simulink model "non_linear_model_2021b"  (R2021b)
settings: Solver=VariableStepAuto  StartTime=0.0  StopTime=8  MaxStep=1e-4  RelTol=1e-7
values from neighbouring files (symbols this model uses):
  beta = 20    [main.m]
undefined symbols (not defined in the file or in its folder): initial_conds, pod
libraries: shared6dof x1
settings Model: Creator=Ferran  LastModifiedBy=ferrandeandres

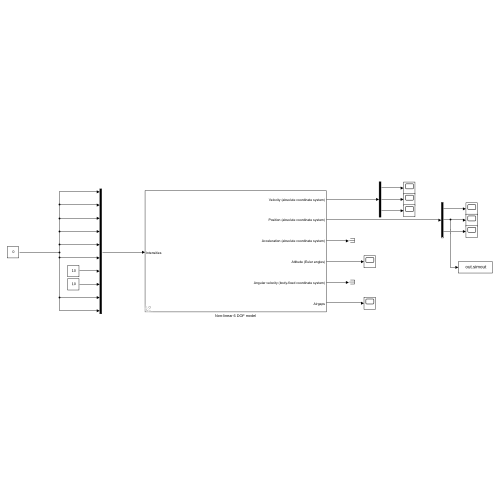
[thumbnail: Simulink's stored preview of the top-level diagram]
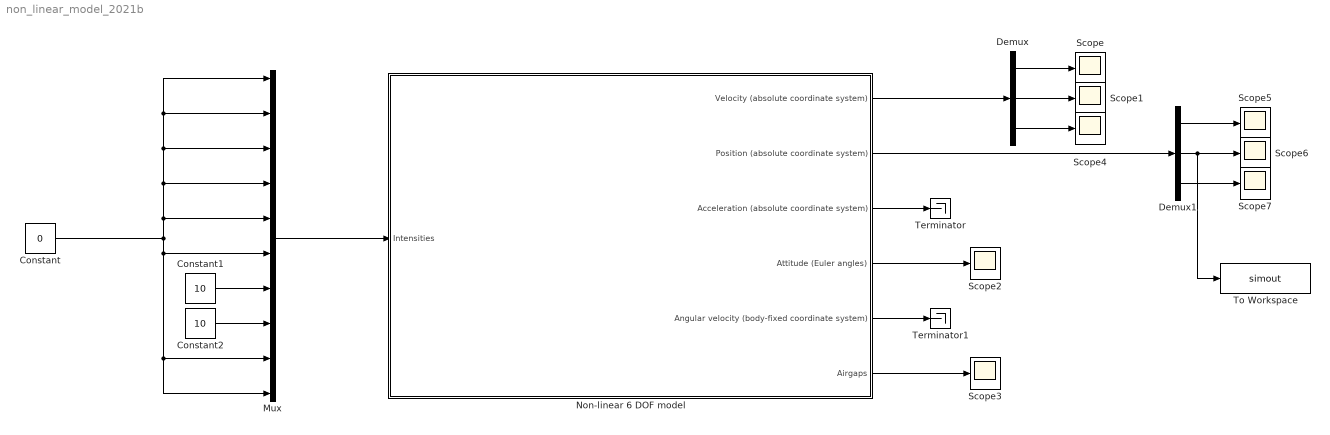
== system non_linear_model_2021b ==
  Constant : Constant  Value=0
  Constant1 : Constant  Value=10
  Constant2 : Constant  Value=10
  Demux : Demux  Outputs=3
  Demux1 : Demux  Outputs=3
  Mux : Mux  Inputs=10
  Non-linear 6 DOF model : Subsystem  AncestorBlock=libH7_6DOF/Non-linear 6 DOF model
  Scope{,1..7} (8 alike) : Scope
  Terminator : Terminator
  Terminator1 : Terminator
  To Workspace : ToWorkspace  VariableName=simout  SaveFormat=Timeseries  SampleTime=-1
  wires:
  Mux/1 -> Non-linear 6 DOF model/1(Intensities)
  Constant/1 -> Mux/4, Mux/2, Mux/1, Mux/3, Mux/5, Mux/6, Mux/9, Mux/10
  Non-linear 6 DOF model/4(Attitude (Euler angles)) -> Scope2/1
  Non-linear 6 DOF model/6(Airgaps) -> Scope3/1
  Non-linear 6 DOF model/3(Acceleration (absolute coordinate system)) -> Terminator/1
  Non-linear 6 DOF model/5(Angular velocity (body-fixed coordinate system)) -> Terminator1/1
  Non-linear 6 DOF model/1(Velocity (absolute coordinate system)) -> Demux/1
  Non-linear 6 DOF model/2(Position (absolute coordinate system)) -> Demux1/1
  Demux/1 -> Scope/1
  Demux/2 -> Scope1/1
  Demux/3 -> Scope4/1
  Demux1/1 -> Scope5/1
  Demux1/2 -> To Workspace/1, Scope6/1
  Demux1/3 -> Scope7/1
  Constant1/1 -> Mux/7
  Constant2/1 -> Mux/8

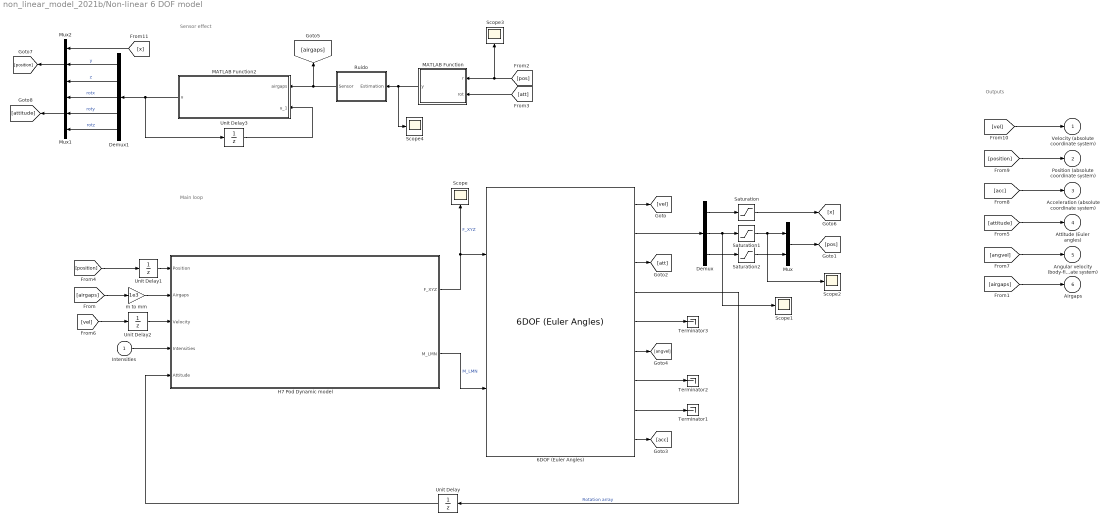
== system non_linear_model_2021b/Non-linear 6 DOF model ==
  note: Outputs
  note: Main loop
  note: Sensor effect
  Intensities : Inport
  6DOF (Euler Angles) : shared6dof/6DOF (Euler Angles)  units=Metric (MKS)  mtype=Fixed  rep=Euler Angles  xme_0=initial_conds.x_0  Vm_0=initial_conds.v_0  eul_0=initial_conds.ang_0  pm_0=initial_conds.w_0  mass_0=pod.mass.mass  mass_e=0.5  mass_f=2.0  inertia=pod.mass.inertia  inertia_e=eye(3)  inertia_f=2*eye(3)  k_quat=1.0  vre_flag=on  abi_flag=on  aMode=0  xme_statename=''  Vm_statename=''  eul_statename=''  quat_statename=''  pm_statename=''  mass_statename=''
      link override Abi: Port=9
      settings: SourceProductBaseCode=AE,PW,DR,MT,VE
  Demux : Demux  Outputs=3
  Demux1 : Demux  Outputs=5
  H7 Pod Dynamic model : Subsystem  AncestorBlock=libH7_6DOF/H7 Pod Dynamic model
      mask Display: image('FBD.png', [0.12 0.12 0.78 0.78]); % Use "Edit Image" on toolstrip to change.
  MATLAB Function : MATLAB Function  TreatAsAtomicUnit=on
  MATLAB Function2 : MATLAB Function  TreatAsAtomicUnit=on
  Mux : Mux  Inputs=2
  Mux1 : Mux  Inputs=3
  Mux2 : Mux  Inputs=3
  Ruido : Subsystem
  Saturation : Saturate  UpperLimit=20  LowerLimit=0
  Saturation1 : Saturate  UpperLimit=0.002  LowerLimit=-0.002
  Saturation2 : Saturate  UpperLimit=0.3504  LowerLimit=0.3384
  Scope{,1..4} (5 alike) : Scope
  Terminator1 : Terminator
  Terminator2 : Terminator
  Terminator3 : Terminator
  Unit Delay : UnitDelay  InitialCondition=eye(3,3)  SampleTime=-1  HasFrameUpgradeWarning=on
  Unit Delay1 : UnitDelay  InitialCondition=initial_conds.x_0  SampleTime=-1  HasFrameUpgradeWarning=on
  Unit Delay2 : UnitDelay  InitialCondition=initial_conds.v_0  SampleTime=-1  HasFrameUpgradeWarning=on
  Unit Delay3 : UnitDelay  SampleTime=-1  HasFrameUpgradeWarning=on
  m to mm : Gain  Gain=1e3
  Velocity (absolute coordinate system) : Outport
  Position (absolute coordinate system) : Outport  Port=2
  Acceleration (absolute coordinate system) : Outport  Port=3
  Attitude (Euler angles) : Outport  Port=4
  Angular velocity (body-fixed coordinate system) : Outport  Port=5
  Airgaps : Outport  Port=6
  wires:
  6DOF (Euler Angles)/7 -> Terminator2/1
  6DOF (Euler Angles)/5 -> Terminator3/1
  6DOF (Euler Angles)/8 -> Terminator1/1
  H7 Pod Dynamic model/2(M_LMN) -> 6DOF (Euler Angles)/2  "M_LMN"
  H7 Pod Dynamic model/1(F_XYZ) -> Scope/1, 6DOF (Euler Angles)/1  "F_XYZ"
  6DOF (Euler Angles)/4 -> Unit Delay/1  "Rotation array"
  Intensities/1 -> H7 Pod Dynamic model/4(Intensities)
  [vel] -> Velocity (absolute coordinate system)/1
  [attitude] -> Attitude (Euler angles)/1
  [angvel] -> Angular velocity (body-fixed coordinate system)/1
  [acc] -> Acceleration (absolute coordinate system)/1
  [position] -> Position (absolute coordinate system)/1
  [airgaps] -> Airgaps/1
  Unit Delay/1 -> H7 Pod Dynamic model/5(Attitude)
  Unit Delay1/1 -> H7 Pod Dynamic model/1(Position)
  [airgaps] -> m to mm/1
  Demux/2 -> Scope1/1, Saturation1/1
  Demux/1 -> Saturation/1
  6DOF (Euler Angles)/2 -> Demux/1
  Demux/3 -> Saturation2/1
  6DOF (Euler Angles)/3 -> [att]
  6DOF (Euler Angles)/1 -> [vel]
  6DOF (Euler Angles)/9 -> [acc]
  6DOF (Euler Angles)/6 -> [angvel]
  [pos] -> Scope3/1, MATLAB Function/1(r)
  [att] -> MATLAB Function/2(rot)
  MATLAB Function/1(y) -> Scope4/1, Ruido/1(Estimation)
  Ruido/1(Sensor) -> MATLAB Function2/1(airgaps), [airgaps]
  [position] -> Unit Delay1/1
  MATLAB Function2/1(u) -> Demux1/1, Unit Delay3/1
  Unit Delay3/1 -> MATLAB Function2/2(u_1)
  Mux/1 -> [pos]
  Saturation/1 -> [x]
  Demux1/3 -> Mux1/1  "rotx"
  Demux1/2 -> Mux2/3  "z"
  Demux1/5 -> Mux1/3  "rotz"
  Demux1/1 -> Mux2/2  "y"
  Demux1/4 -> Mux1/2  "roty"
  [x] -> Mux2/1
  Mux2/1 -> [position]
  Mux1/1 -> [attitude]
  [vel] -> Unit Delay2/1
  Unit Delay2/1 -> H7 Pod Dynamic model/3(Velocity)
  Saturation1/1 -> Scope2/1, Mux/1
  Saturation2/1 -> Mux/2
  m to mm/1 -> H7 Pod Dynamic model/2(Airgaps)

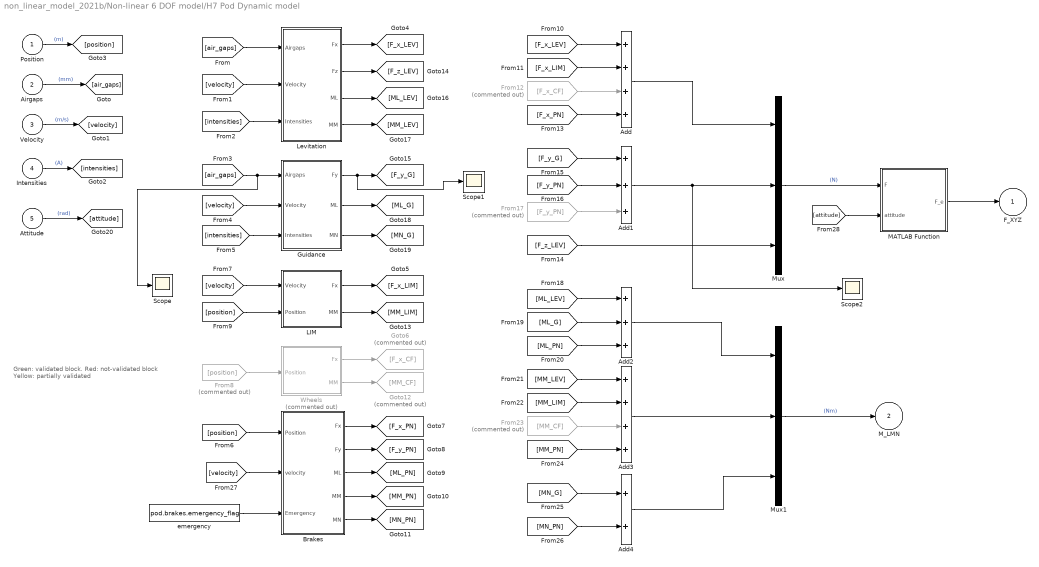
== system non_linear_model_2021b/Non-linear 6 DOF model/H7 Pod Dynamic model ==
  note: Green: validated block.
      | Red: not-validated block
      | Yellow: partially validated
  Position : Inport
  Airgaps : Inport  Port=2
  Velocity : Inport  Port=3
  Intensities : Inport  Port=4
  Attitude : Inport  Port=5
  Add : Sum  Inputs=++++
  Add1 : Sum  Inputs=+++
  Add2 : Sum  Inputs=+++
  Add3 : Sum  Inputs=++++
  Add4 : Sum
  Brakes : Subsystem
  From12 : From  Commented=on  GotoTag=F_x_CF
  From17 : From  Commented=on  GotoTag=F_y_PN
  From23 : From  Commented=on  GotoTag=MM_CF
  From8 : From  Commented=on  GotoTag=position
  Goto12 : Goto  Commented=on  GotoTag=MM_CF
  Goto6 : Goto  Commented=on  GotoTag=F_x_CF
  Guidance : Subsystem
  LIM : Subsystem
  Levitation : Subsystem
  MATLAB Function : MATLAB Function  TreatAsAtomicUnit=on
  Mux : Mux  Inputs=3
  Mux1 : Mux  Inputs=3
  Scope : Scope
  Scope1 : Scope
  Scope2 : Scope
  Wheels : Subsystem  Commented=on
  emergency : Constant  Value=pod.brakes.emergency_flag
  F_XYZ : Outport
  M_LMN : Outport  Port=2
  wires:
  MATLAB Function/1(F_e) -> F_XYZ/1
  [attitude] -> MATLAB Function/2(attitude)
  Attitude/1 -> [attitude]  "(rad)"
  [velocity] -> Brakes/2(velocity)
  Add4/1 -> Mux1/3
  [MN_G] -> Add4/1
  [MN_PN] -> Add4/2
  From23/1 -> Add3/3
  [MM_LIM] -> Add3/2
  Add3/1 -> Mux1/2
  [MM_PN] -> Add3/4
  [MM_LEV] -> Add3/1
  [ML_PN] -> Add2/3
  [ML_G] -> Add2/2
  Add2/1 -> Mux1/1
  [ML_LEV] -> Add2/1
  Add1/1 -> Scope2/1, Mux/2
  From17/1 -> Add1/3
  [F_y_PN] -> Add1/2
  [F_y_G] -> Add1/1
  [F_z_LEV] -> Mux/3
  [F_x_PN] -> Add/4
  From12/1 -> Add/3
  [F_x_LIM] -> Add/2
  [F_x_LEV] -> Add/1
  Add/1 -> Mux/1
  Guidance/3(MN) -> [MN_G]
  Guidance/2(ML) -> [ML_G]
  Levitation/4(MM) -> [MM_LEV]
  Levitation/3(ML) -> [ML_LEV]
  Guidance/1(Fy) -> Scope1/1, [F_y_G]
  Levitation/2(Fz) -> [F_z_LEV]
  LIM/2(MM) -> [MM_LIM]
  Wheels/2(MM) -> Goto12/1
  Brakes/5(MN) -> [MN_PN]
  Brakes/4(MM) -> [MM_PN]
  Brakes/3(ML) -> [ML_PN]
  Brakes/2(Fy) -> [F_y_PN]
  Brakes/1(Fx) -> [F_x_PN]
  Wheels/1(Fx) -> Goto6/1
  LIM/1(Fx) -> [F_x_LIM]
  Levitation/1(Fx) -> [F_x_LEV]
  [position] -> LIM/2(Position)
  From8/1 -> Wheels/1(Position)
  emergency/1 -> Brakes/3(Emergency)
  [position] -> Brakes/1(Position)
  Position/1 -> [position]  "(m)"
  [velocity] -> LIM/1(Velocity)
  [air_gaps] -> Scope/1, Guidance/1(Airgaps)
  [intensities] -> Guidance/3(Intensities)
  [velocity] -> Guidance/2(Velocity)
  [intensities] -> Levitation/3(Intensities)
  [velocity] -> Levitation/2(Velocity)
  [air_gaps] -> Levitation/1(Airgaps)
  Mux1/1 -> M_LMN/1  "(Nm)"
  Mux/1 -> MATLAB Function/1(F)  "(N)"
  Intensities/1 -> [intensities]  "(A)"
  Velocity/1 -> [velocity]  "(m/s)"
  Airgaps/1 -> [air_gaps]  "(mm)"

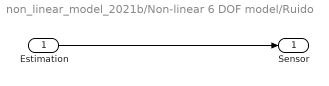
== system non_linear_model_2021b/Non-linear 6 DOF model/Ruido ==
  Estimation : Inport
  Sensor : Outport
  wires:
  Estimation/1 -> Sensor/1

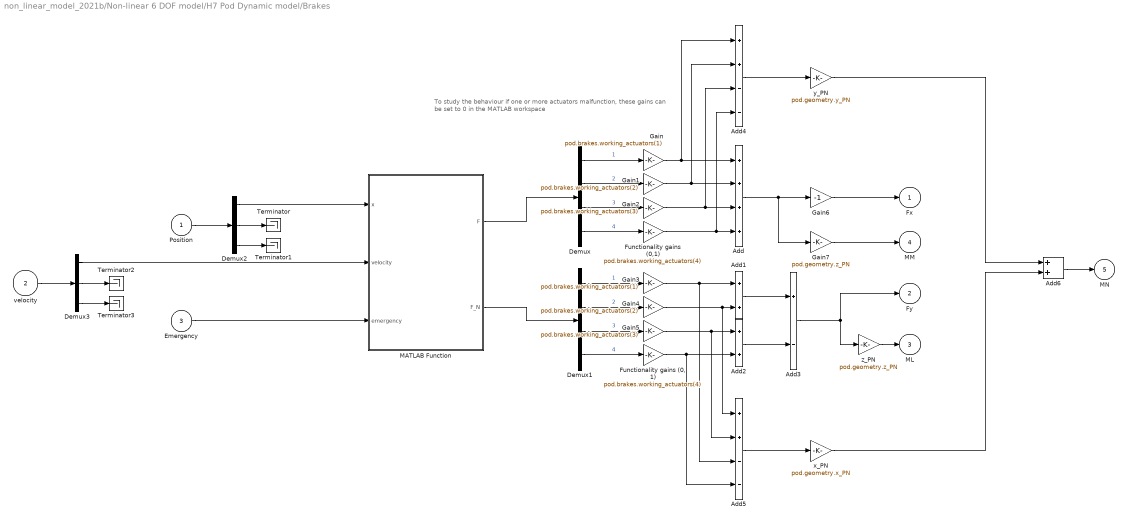
== system non_linear_model_2021b/Non-linear 6 DOF model/H7 Pod Dynamic model/Brakes ==
  note: To study the behaviour if one or more actuators malfunction,
      | these gains can be set to 0 in the MATLAB workspace
  Position : Inport
  velocity : Inport  Port=2
  Emergency : Inport  Port=3
  Add : Sum  Inputs=++++
  Add1 : Sum
  Add2 : Sum
  Add3 : Sum  Inputs=+-
  Add4 : Sum  Inputs=++--
  Add5 : Sum  Inputs=++--
  Add6 : Sum
  Demux : Demux
  Demux1 : Demux
  Demux2 : Demux  Outputs=3
  Demux3 : Demux  Outputs=3
  "Functionality gains (0, 1)" : Gain  Gain=pod.brakes.working_actuators(4)
  Functionality gains (0,1) : Gain  Gain=pod.brakes.working_actuators(4)
  Gain : Gain  Gain=pod.brakes.working_actuators(1)
  Gain1 : Gain  Gain=pod.brakes.working_actuators(2)
  Gain2 : Gain  Gain=pod.brakes.working_actuators(3)
  Gain3 : Gain  Gain=pod.brakes.working_actuators(1)
  Gain4 : Gain  Gain=pod.brakes.working_actuators(2)
  Gain5 : Gain  Gain=pod.brakes.working_actuators(3)
  Gain6 : Gain  Gain=-1
  Gain7 : Gain  Gain=pod.geometry.z_PN
  MATLAB Function : MATLAB Function  TreatAsAtomicUnit=on
  Terminator{,1..3} (4 alike) : Terminator
  x_PN : Gain  Gain=pod.geometry.x_PN
  y_PN : Gain  Gain=pod.geometry.y_PN
  z_PN : Gain  Gain=pod.geometry.z_PN
  Fx : Outport
  Fy : Outport  Port=2
  ML : Outport  Port=3
  MM : Outport  Port=4
  MN : Outport  Port=5
  wires:
  x_PN/1 -> Add6/2
  y_PN/1 -> Add6/1
  Add6/1 -> MN/1
  Add5/1 -> x_PN/1
  Demux3/1 -> MATLAB Function/2(velocity)
  Demux3/3 -> Terminator3/1
  Demux3/2 -> Terminator2/1
  velocity/1 -> Demux3/1
  Demux2/2 -> Terminator/1
  Demux2/1 -> MATLAB Function/1(x)
  Position/1 -> Demux2/1
  Demux2/3 -> Terminator1/1
  Add4/1 -> y_PN/1
  Gain7/1 -> MM/1
  z_PN/1 -> ML/1
  Add3/1 -> Fy/1, z_PN/1
  Add2/1 -> Add3/2
  Add1/1 -> Add3/1
  "Functionality gains (0, 1)"/1 -> Add5/4, Add2/2
  Gain5/1 -> Add2/1, Add5/2
  Gain3/1 -> Add5/3, Add1/1
  Gain4/1 -> Add1/2, Add5/1
  Gain6/1 -> Fx/1
  Add/1 -> Gain6/1, Gain7/1
  Gain/1 -> Add/1, Add4/1
  Gain1/1 -> Add/2, Add4/2
  Gain2/1 -> Add/3, Add4/3
  Functionality gains (0,1)/1 -> Add/4, Add4/4
  MATLAB Function/2(F_N) -> Demux1/1
  Demux1/2 -> Gain4/1  "2"
  Demux1/1 -> Gain3/1  "1"
  Demux1/3 -> Gain5/1  "3"
  Demux1/4 -> "Functionality gains (0, 1)"/1  "4"
  Demux/4 -> Functionality gains (0,1)/1  "4"
  Demux/3 -> Gain2/1  "3"
  Demux/2 -> Gain1/1  "2"
  Demux/1 -> Gain/1  "1"
  MATLAB Function/1(F) -> Demux/1
  Emergency/1 -> MATLAB Function/3(emergency)

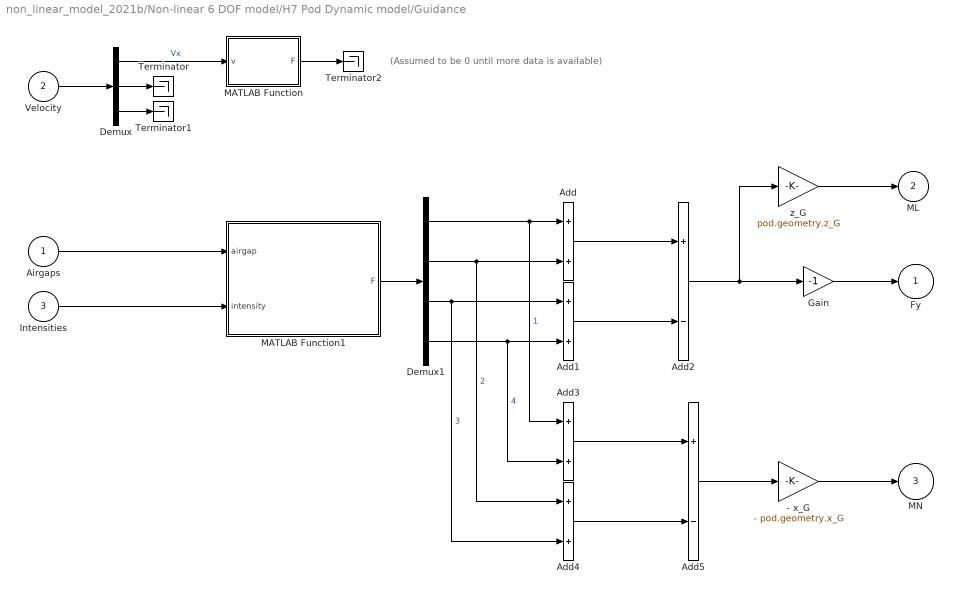
== system non_linear_model_2021b/Non-linear 6 DOF model/H7 Pod Dynamic model/Guidance ==
  note: (Assumed to be 0 until more data is available)
  Airgaps : Inport
  Velocity : Inport  Port=2
  Intensities : Inport  Port=3
  - x_G : Gain  Gain=- pod.geometry.x_G
  Add{,1,3..4} (4 alike) : Sum
  Add2 : Sum  Inputs=+-
  Add5 : Sum  Inputs=+-
  Demux : Demux  Outputs=3
  Demux1 : Demux
  Gain : Gain  Gain=-1
  MATLAB Function : MATLAB Function  TreatAsAtomicUnit=on
  MATLAB Function1 : MATLAB Function  TreatAsAtomicUnit=on
  Terminator : Terminator
  Terminator1 : Terminator
  Terminator2 : Terminator
  z_G : Gain  Gain=pod.geometry.z_G
  Fy : Outport
  ML : Outport  Port=2
  MN : Outport  Port=3
  wires:
  - x_G/1 -> MN/1
  Add5/1 -> - x_G/1
  Add4/1 -> Add5/2
  Add3/1 -> Add5/1
  z_G/1 -> ML/1
  Add2/1 -> Gain/1, z_G/1
  Add/1 -> Add2/1
  Add1/1 -> Add2/2
  Demux1/4 -> Add1/2, Add3/2  "4"
  Demux1/3 -> Add1/1, Add4/2  "3"
  Demux1/2 -> Add/2, Add4/1  "2"
  Demux1/1 -> Add/1, Add3/1  "1"
  Airgaps/1 -> MATLAB Function1/1(airgap)
  Intensities/1 -> MATLAB Function1/2(intensity)
  MATLAB Function1/1(F) -> Demux1/1
  MATLAB Function/1(F) -> Terminator2/1
  Demux/3 -> Terminator1/1
  Demux/2 -> Terminator/1
  Velocity/1 -> Demux/1
  Demux/1 -> MATLAB Function/1(v)  "Vx"
  Gain/1 -> Fy/1

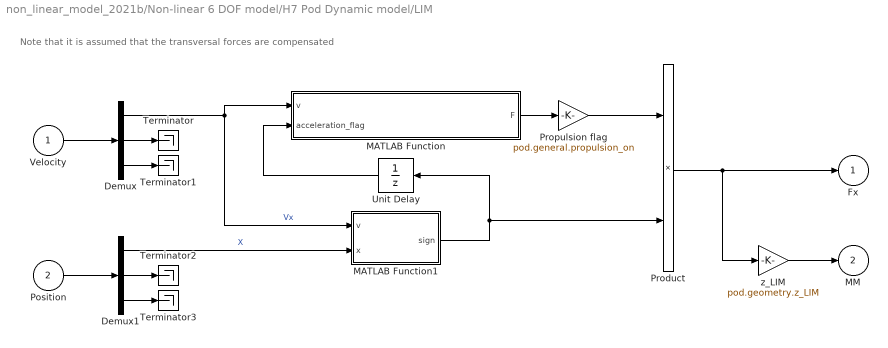
== system non_linear_model_2021b/Non-linear 6 DOF model/H7 Pod Dynamic model/LIM ==
  note: Note that it is assumed that the transversal forces are compensated
  Velocity : Inport
  Position : Inport  Port=2
  Demux : Demux  Outputs=3
  Demux1 : Demux  Outputs=3
  MATLAB Function : MATLAB Function  TreatAsAtomicUnit=on
  MATLAB Function1 : MATLAB Function  TreatAsAtomicUnit=on
  Product : Product
  Propulsion flag : Gain  Gain=pod.general.propulsion_on
  Terminator{,1..3} (4 alike) : Terminator
  Unit Delay : UnitDelay  InitialCondition=1  SampleTime=-1  HasFrameUpgradeWarning=on
  z_LIM : Gain  Gain=pod.geometry.z_LIM
  Fx : Outport
  MM : Outport  Port=2
  wires:
  z_LIM/1 -> MM/1
  Product/1 -> Fx/1, z_LIM/1
  MATLAB Function/1(F) -> Propulsion flag/1
  MATLAB Function1/1(sign) -> Unit Delay/1, Product/2
  Demux1/1 -> MATLAB Function1/2(x)  "X"
  Demux1/2 -> Terminator2/1
  Demux1/3 -> Terminator3/1
  Position/1 -> Demux1/1
  Demux/1 -> MATLAB Function/1(v), MATLAB Function1/1(v)  "Vx"
  Demux/3 -> Terminator1/1
  Demux/2 -> Terminator/1
  Velocity/1 -> Demux/1
  Propulsion flag/1 -> Product/1
  Unit Delay/1 -> MATLAB Function/2(acceleration_flag)

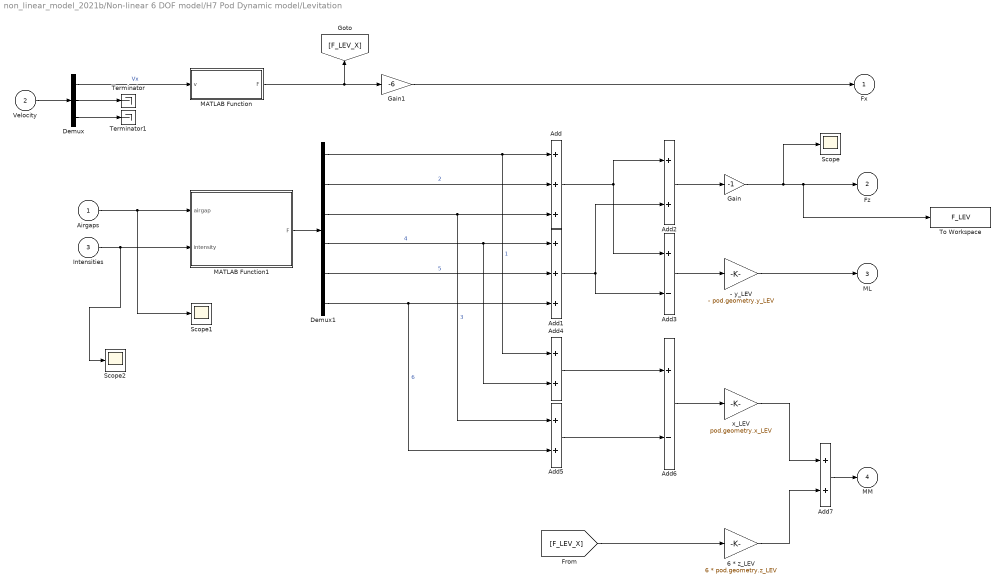
== system non_linear_model_2021b/Non-linear 6 DOF model/H7 Pod Dynamic model/Levitation ==
  Airgaps : Inport
  Velocity : Inport  Port=2
  Intensities : Inport  Port=3
  - y_LEV : Gain  Gain=- pod.geometry.y_LEV
  6 * z_LEV : Gain  Gain=6 * pod.geometry.z_LEV
  Add : Sum  Inputs=+++
  Add1 : Sum  Inputs=+++
  Add{2,4..5,7} (4 alike) : Sum
  Add3 : Sum  Inputs=+-
  Add6 : Sum  Inputs=+-
  Demux : Demux  Outputs=3
  Demux1 : Demux  Outputs=6
  Gain : Gain  Gain=-1
  Gain1 : Gain  Gain=-6
  MATLAB Function : MATLAB Function  TreatAsAtomicUnit=on
  MATLAB Function1 : MATLAB Function  TreatAsAtomicUnit=on
  Scope : Scope
  Scope1 : Scope
  Scope2 : Scope
  Terminator : Terminator
  Terminator1 : Terminator
  To Workspace : ToWorkspace  VariableName=F_LEV  SaveFormat=Timeseries  SampleTime=-1
  x_LEV : Gain  Gain=pod.geometry.x_LEV
  Fx : Outport
  Fz : Outport  Port=2
  ML : Outport  Port=3
  MM : Outport  Port=4
  wires:
  MATLAB Function/1(F) -> Gain1/1, [F_LEV_X]
  6 * z_LEV/1 -> Add7/2
  x_LEV/1 -> Add7/1
  Add7/1 -> MM/1
  Add6/1 -> x_LEV/1
  Add5/1 -> Add6/2
  Add4/1 -> Add6/1
  [F_LEV_X] -> 6 * z_LEV/1
  Gain1/1 -> Fx/1
  - y_LEV/1 -> ML/1
  Add3/1 -> - y_LEV/1
  Add2/1 -> Gain/1
  Add1/1 -> Add3/2, Add2/2
  Add/1 -> Add3/1, Add2/1
  Demux1/6 -> Add1/3, Add5/2  "6"
  Demux1/5 -> Add1/2  "5"
  Demux1/4 -> Add1/1, Add4/2  "4"
  Demux1/3 -> Add/3, Add5/1  "3"
  Demux1/2 -> Add/2  "2"
  Demux1/1 -> Add/1, Add4/1  "1"
  Gain/1 -> Scope/1, To Workspace/1, Fz/1
  MATLAB Function1/1(F) -> Demux1/1
  Intensities/1 -> Scope2/1, MATLAB Function1/2(intensity)
  Airgaps/1 -> Scope1/1, MATLAB Function1/1(airgap)
  Demux/1 -> MATLAB Function/1(v)  "Vx"
  Velocity/1 -> Demux/1
  Demux/3 -> Terminator1/1
  Demux/2 -> Terminator/1

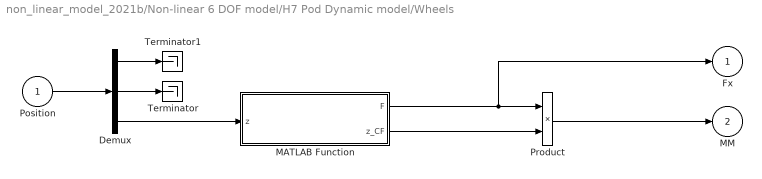
== system non_linear_model_2021b/Non-linear 6 DOF model/H7 Pod Dynamic model/Wheels ==
  Position : Inport
  Demux : Demux  Outputs=3
  MATLAB Function : MATLAB Function  TreatAsAtomicUnit=on
  Product : Product
  Terminator : Terminator
  Terminator1 : Terminator
  Fx : Outport
  MM : Outport  Port=2
  wires:
  Product/1 -> MM/1
  MATLAB Function/2(z_CF) -> Product/2
  Demux/1 -> Terminator1/1
  MATLAB Function/1(F) -> Product/1, Fx/1
  Demux/3 -> MATLAB Function/1(z)
  Demux/2 -> Terminator/1
  Position/1 -> Demux/1

== matlab function non_linear_model_2021b/Non-linear 6 DOF model/MATLAB Function2 ==
  data: airgaps input; u_1 input; u output; pod parameter; beta parameter
function u  = ag2pos(airgaps, u_1, pod, beta)
% Computes the position and attitute od the pod as a function of the airgaps 
% ═════════════════════════════════════════════════════════════════════════
% Last updated: 27.01.2022
% ═════════════════════════════════════════════════════════════════════════
% INPUT:
%   airgaps   = Vector with airgaps in [m]. The 6 first values correspond
%               to the levitation units, and the 4 last values correspond 
%               to guidance. 
%               Size 10 x 1
%   beta      = Measure acceptance tolerance [-]
%               Scalar
%   pod       = Struct containing data about
%                   *mass (Mass and inertia)
%                   *brakes (Pressures, friction coefficients and forces)
%                   *levitation (Maps of forces)
%                   *guiding (Maps of forces)
%                   *propulsion (Force as a function of velocity). 
%                   *geometry (points of application of forces wrt CG)
%                   *general (simulation parameters)
%   u         = DOF vector in (t-1), containing the estimations of the 
%               position in the y and z directions [m] and the 3 rotation 
%               angles [rad]
%               Size 5 x 1
% OUTPUT:
%   u         = DOF vector, containing the estimations of the position in
%               the y and z directions [m] and the 3 rotation angles [rad]
%               Size 5 x 1
% ═════════════════════════════════════════════════════════════════════════


%%% Input check (4 inputs)
narginchk(4,4);

%%% Ensure inputs are well defined
% airgaps must be a 10 dimensional vector
if ~ismatrix(airgaps) || numel(airgaps) ~= 10
    error('Vector with airgaps is not properly defined');
end

% % Filter incorrect measures
% if any(isnan(airgaps))
%     warning('Signal of unit number %d is incorrect. The system will ignore it, but computation will be slower.', find(isnan(airgaps)));
%     airgaps(isnan(airgaps)) = 0;
% end

% % Beta must be scalar
% if ~(isscalar(beta))
%     error('beta must be an scalar')
% end


%%% Auxiliar vectors initialization 
coder.varsize('y_aux'); 
coder.varsize('z_aux'); 
coder.varsize('rotx_aux');
coder.varsize('roty_aux');
coder.varsize('rotz_aux')
coder.varsize('malfunction'); 

y_aux       = zeros(4,1);
idx_y       = false(4,1);
z_aux       = zeros(6,1);
idx_z       = false(6,1);
rotx_aux    = zeros(3,1);
idxx        = false(3,1);
roty_aux    = zeros(6,1);
idxy        = false(6,1);
rotz_aux    = zeros(2,1);
idxz        = false(2,1);
malfunction = true(11,1);
y = 0; z = 0; rotx = 0; roty = 0; rotz = 0;

%%% Attitude
rotx_aux(1) = asin((airgaps(1) - airgaps(4))/(2 * pod.geometry.y_LEV));
rotx_aux(2) = asin((airgaps(2) - airgaps(5))/(2 * pod.geometry.y_LEV));
rotx_aux(3) = asin((airgaps(3) - airgaps(6))/(2 * pod.geometry.y_LEV));

roty_aux(1) = asin((airgaps(5) - airgaps(4))/(    pod.geometry.z_LEV));
roty_aux(2) = asin((airgaps(6) - airgaps(4))/(2 * pod.geometry.z_LEV));
roty_aux(3) = asin((airgaps(6) - airgaps(5))/(    pod.geometry.z_LEV));
roty_aux(4) = asin((airgaps(3) - airgaps(2))/(    pod.geometry.z_LEV));
roty_aux(5) = asin((airgaps(3) - airgaps(1))/(2 * pod.geometry.z_LEV));
roty_aux(6) = asin((airgaps(2) - airgaps(1))/(    pod.geometry.z_LEV));

rotz_aux(1) = asin((airgaps(8) - airgaps(7 ))/(2 * pod.geometry.x_G));
rotz_aux(1) = asin((airgaps(9) - airgaps(10))/(2 * pod.geometry.x_G));

while any(malfunction)
    rotx = mean(rotx_aux);
    roty = mean(roty_aux);
    rotz = mean(rotz_aux);

    resx = abs(rotx_aux - rotx);
    resy = abs(roty_aux - roty);
    resz = abs(rotz_aux - rotz);

    idxx =  (resx> abs(beta*rotx));
    idxy =  (resy> abs(beta*roty));
    idxz =  (resz> abs(beta*rotz));

    malfunction = [idxx; idxy; idxz];

    rotx_aux = rotx_aux(~(idxx));
    roty_aux = roty_aux(~(idxy));
    rotz_aux = rotz_aux(~(idxz));
end

malfunction = true(10,1);

%%% Position
y_aux(1) = airgaps(7)  + pod.geometry.y_G * cos(rotz) + pod.geometry.x_G * sin(rotz);
y_aux(2) = airgaps(8)  + pod.geometry.y_G * cos(rotz) - pod.geometry.x_G * sin(rotz);
y_aux(3) = - airgaps(9)  - pod.geometry.y_G * cos(rotz) - pod.geometry.x_G * sin(rotz);
y_aux(4) = - airgaps(10) - pod.geometry.y_G * cos(rotz) + pod.geometry.x_G * sin(rotz);

z_aux(1) = airgaps(1)  + pod.geometry.z_LEV * cos(roty) + pod.geometry.x_LEV * sin(roty) - pod.geometry.y_LEV * sin(rotx);
z_aux(2) = airgaps(2)  + pod.geometry.z_LEV * cos(roty)                                  - pod.geometry.y_LEV * sin(rotx);
z_aux(3) = airgaps(3)  + pod.geometry.z_LEV * cos(roty) - pod.geometry.x_LEV * sin(roty) - pod.geometry.y_LEV * sin(rotx);
z_aux(4) = airgaps(4)  + pod.geometry.z_LEV * cos(roty) + pod.geometry.x_LEV * sin(roty) + pod.geometry.y_LEV * sin(rotx);
z_aux(5) = airgaps(5)  + pod.geometry.z_LEV * cos(roty)                                  + pod.geometry.y_LEV * sin(rotx);
z_aux(6) = airgaps(6)  + pod.geometry.z_LEV * cos(roty) - pod.geometry.x_LEV * sin(roty) + pod.geometry.y_LEV * sin(rotx);


while any(malfunction)
    y = mean(y_aux);
    z = mean(z_aux);

    resy = abs(y_aux - y);
    resz = abs(z_aux - z);

    idx_y = (resy>beta*y);
    idx_z = (resz>beta*z);

    malfunction = [idxy; idxz];

    y_aux = y_aux(~(idx_y));
    z_aux = z_aux(~(idx_z));
end

u = [y, z, rotx, roty, rotz]';

u(isnan(u)) = u_1(isnan(u));

end

== matlab function non_linear_model_2021b/Non-linear 6 DOF model/MATLAB Function ==
  data: r input; y output; rot input; pod parameter
function y = pos2ag3D(r, rot, pod)
% Computes the airgaps as a function of the position and the attitude
% ═════════════════════════════════════════════════════════════════════════
% Last updated: 02.02.2022
% ═════════════════════════════════════════════════════════════════════════

y_CG  = r(1);
z_CG  = r(2);
rot_x = rot(1);
rot_y = rot(2);
rot_z = rot(3); 

AG_0  = 10e-3;

AG_1 = z_CG  -  pod.geometry.z_LEV * cos(rot_y)  -  pod.geometry.x_LEV * sin(rot_y)  +  pod.geometry.y_LEV * sin(rot_x);
AG_2 = z_CG  -  pod.geometry.z_LEV * cos(rot_y)                                      +  pod.geometry.y_LEV * sin(rot_x);
AG_3 = z_CG  -  pod.geometry.z_LEV * cos(rot_y)  +  pod.geometry.x_LEV * sin(rot_y)  +  pod.geometry.y_LEV * sin(rot_x);
AG_4 = z_CG  -  pod.geometry.z_LEV * cos(rot_y)  -  pod.geometry.x_LEV * sin(rot_y)  -  pod.geometry.y_LEV * sin(rot_x);
AG_5 = z_CG  -  pod.geometry.z_LEV * cos(rot_y)                                      -  pod.geometry.y_LEV * sin(rot_x);
AG_6 = z_CG  -  pod.geometry.z_LEV * cos(rot_y)  +  pod.geometry.x_LEV * sin(rot_y)  -  pod.geometry.y_LEV * sin(rot_x);

AG_7  =   y_CG  - pod.geometry.x_G * sin(rot_z) + AG_0;
AG_8  =   y_CG  + pod.geometry.x_G * sin(rot_z) + AG_0;
AG_9  = - y_CG  + pod.geometry.x_G * sin(rot_z) + AG_0;  
AG_10 = - y_CG  - pod.geometry.x_G * sin(rot_z) + AG_0; 

y = [AG_1; AG_2; AG_3; AG_4; AG_5; AG_6; AG_7; AG_8; AG_9; AG_10];

y(y<0) = 0;

== matlab function non_linear_model_2021b/Non-linear 6 DOF model/H7 Pod Dynamic model/Levitation/MATLAB Function ==
  data: v input; F output; pod parameter
function F = HEMSdrag(v, pod)
% Computes the drag force (N) of one HEMS unit as a function of the 
% velocity (m/s)
% ═════════════════════════════════════════════════════════════════════════
% Last updated: 15.12.2021
% ═════════════════════════════════════════════════════════════════════════

F = pod.levitation.drag_1_unit.poly.p3*v^3 + ...
    pod.levitation.drag_1_unit.poly.p2*v^2 + ...
    pod.levitation.drag_1_unit.poly.p1*v   ;

== matlab function non_linear_model_2021b/Non-linear 6 DOF model/H7 Pod Dynamic model/Guidance/MATLAB Function ==
  data: v input; F output
function F = EMSdrag(v)
% Computes the drag force (N) of one EMS units as a function of 
% its velocity (m/s)
% ═════════════════════════════════════════════════════════════════════════
% Last updated: 15.12.2021
% ════════════════════════════════════════════════════════════════════════

F = 0;

== matlab function non_linear_model_2021b/Non-linear 6 DOF model/H7 Pod Dynamic model/Guidance/MATLAB Function1 ==
  data: airgap input; F output; intensity input; pod parameter
function F = EMSlev(airgap, intensity, pod)
% Computes the levitation force (N) of all the EMS units as a function of 
% their air gaps (mm) and intensities (A)
% ═════════════════════════════════════════════════════════════════════════
% Last updated: 15.12.2021
% ════════════════════════════════════════════════════════════════════════

x   = airgap(7:10);
y   = intensity(7:10);

F = pod.guiding.poly.p00 + ...
    pod.guiding.poly.p10.*x + ...
    pod.guiding.poly.p01.*y + ...
    pod.guiding.poly.p20.*x.^2 + ...
    pod.guiding.poly.p11.*x.*y + ...
    pod.guiding.poly.p02.*y.^2 + ...
    pod.guiding.poly.p21.*x.^2.*y + ...
    pod.guiding.poly.p12.*x.*y.^2 + ...
    pod.guiding.poly.p03.*y.^3;

== matlab function non_linear_model_2021b/Non-linear 6 DOF model/H7 Pod Dynamic model/LIM/MATLAB Function ==
  data: v input; acceleration_flag input; F output; pod parameter
function F = LIMtraction(v, acceleration_flag, pod)
% Computes the traction force (N) of the LIM as a function of 
% the absolute velocity of the prototype (m/s)
% ═════════════════════════════════════════════════════════════════════════
% Last updated: 20.12.2021
% ═════════════════════════════════════════════════════════════════════════

if acceleration_flag == 1
    F = pod.propulsion.poly.p3*v^3 + ...
        pod.propulsion.poly.p2*v^2 + ...
        pod.propulsion.poly.p1*v   + ...
        pod.propulsion.poly.p0;

else
    F = pod.propulsion.br_poly.p2*v^2 + ...
        pod.propulsion.br_poly.p1*v   + ...
        pod.propulsion.br_poly.p0;
end

== matlab function non_linear_model_2021b/Non-linear 6 DOF model/H7 Pod Dynamic model/LIM/MATLAB Function1 ==
  data: v input; x input; sign output; pod parameter
function sign = LIMdirection(v, x, pod)
% Decides if the LIM force is being applied to accelerate or to brake 
% by comparing the position of the pod with a predefined treshold
% ═════════════════════════════════════════════════════════════════════════
% Last updated: 20.12.2021
% ═════════════════════════════════════════════════════════════════════════

if x >= pod.brakes.d && v > 0    
    sign = -1;
elseif x >= pod.brakes.d && v <= 0
    sign = 0;
else
    sign = 1;
end

== matlab function non_linear_model_2021b/Non-linear 6 DOF model/H7 Pod Dynamic model/Levitation/MATLAB Function1 ==
  data: airgap input; F output; intensity input; pod parameter
function F = HEMSlev(airgap, intensity, pod)
% Computes the levitation force (N) of all the HEMS units as a function of 
% their air gaps (mm) and intensities (A)
% ═════════════════════════════════════════════════════════════════════════
% Last updated: 15.12.2021
% ════════════════════════════════════════════════════════════════════════

x   = airgap(1:6);
y   = intensity(1:6);

F = pod.levitation.poly_1_unit.p00 + ...
    pod.levitation.poly_1_unit.p10.*x + ...
    pod.levitation.poly_1_unit.p01.*y + ...
    pod.levitation.poly_1_unit.p20.*x.^2 + ...
    pod.levitation.poly_1_unit.p11.*x.*y + ...
    pod.levitation.poly_1_unit.p02.*y.^2 + ...
    pod.levitation.poly_1_unit.p21.*x.^2.*y + ...
    pod.levitation.poly_1_unit.p12.*x.*y.^2 + ...
    pod.levitation.poly_1_unit.p03.*y.^3;

== matlab function non_linear_model_2021b/Non-linear 6 DOF model/H7 Pod Dynamic model/MATLAB Function ==
  data: F input; F_e output; attitude input; pod parameter
function F_e = BF2E(F, attitude, pod)
% Computes the total force in absoute axis
% ═════════════════════════════════════════════════════════════════════════
% Last updated: 27.12.2021
% ═════════════════════════════════════════════════════════════════════════
F     = reshape(F, [3 1]);


F_e = attitude * F + pod.mass.mass * [0 0 9.81]';

== matlab function non_linear_model_2021b/Non-linear 6 DOF model/H7 Pod Dynamic model/Wheels/MATLAB Function ==
  data: z input; F output; pod parameter; z_CF output
function [F, z_CF] = rollingFriction(z, pod)
% Computes the rolling resistance force (N) of the wheels. It distinguishes
% 3 cases: 
%   (1) z = 0. Pod touching the ground
%   (2) z = z_max. Pod touching the ceiling. It is assumed no current
%   applied to the HEMS. 
%   (3) Otherwise. Pod levitating. 
% ═════════════════════════════════════════════════════════════════════════
% Last updated: 26.12.2021
% ═════════════════════════════════════════════════════════════════════════

% F_LEV worst case scenario computation
x   = 12; % [mm]
y   = 0;  % [A]

F_LEV = pod.levitation.poly_1_unit.p00 + ...
        pod.levitation.poly_1_unit.p10.*x + ...
        pod.levitation.poly_1_unit.p01.*y + ...
        pod.levitation.poly_1_unit.p20.*x.^2 + ...
        pod.levitation.poly_1_unit.p11.*x.*y + ...
        pod.levitation.poly_1_unit.p02.*y.^2 + ...
        pod.levitation.poly_1_unit.p21.*x.^2.*y + ...
        pod.levitation.poly_1_unit.p12.*x.*y.^2 + ...
        pod.levitation.poly_1_unit.p03.*y.^3;

% Main algorithm
if z == 0
    F_N   = pod.mass.mass * 9.81;
    z_CF  = - pod.geometry.z_CF;
elseif z == pod.general.z_range
    F_N   = 6 * F_LEV - pod.mass.mass * 9.81;
    z_CF  = pod.geometry.z_CF;
else
    F_N   = 0;
    z_CF  = 0;
end

F = pod.wheels.number * pod.wheels.roll_coef * F_N;

== matlab function non_linear_model_2021b/Non-linear 6 DOF model/H7 Pod Dynamic model/Brakes/MATLAB Function ==
  data: x input; velocity input; F output; emergency input; F_N output; pod parameter
function [F, F_N] = brakes_activation(x, velocity, emergency, pod)
% Computes the braking force of the pneumatic actuators if and only if 
%     (1) The emergency flag has been raised
%     (2) The pod is above the acceleration phase distance
% ═════════════════════════════════════════════════════════════════════════
% Last updated: 20.12.2021
% ═════════════════════════════════════════════════════════════════════════

if (emergency == 1 && x >= pod.brakes.d && velocity >= 0)
    F       = pod.brakes.force * ones(pod.brakes.n,1);
    F_N     = pod.brakes.normal_force * ones(pod.brakes.n,1);
else
    F       = zeros(pod.brakes.n,1);
    F_N     = zeros(pod.brakes.n,1);
end
